simulink model "modelTest"  (R2025a)
settings: Solver=ode8  StartTime=0.0  StopTime=1000  FixedStep=0.1  RelTol=1e-3
libraries: simulink x2
settings Model: DataDictionary=Constants.sldd  PacingRate=9  Creator=levirogalla  LastModifiedBy=levirogalla
settings ModelReferenceCC: ModelReferenceMinAlgLoopOccurrences=on

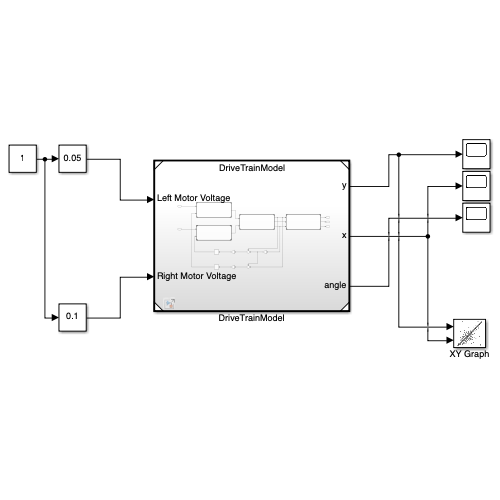
[thumbnail: Simulink's stored preview of the top-level diagram]
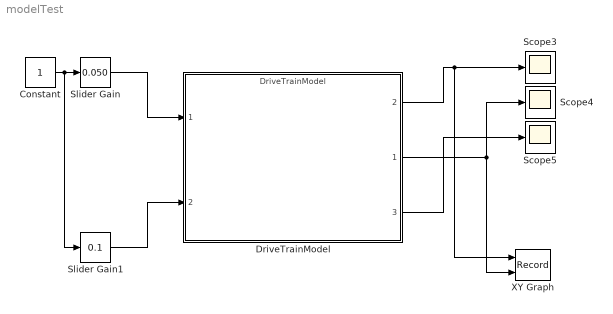
== system modelTest ==
  Constant : Constant
  DriveTrainModel : ModelReference  ModelNameDialog=DriveTrainModel.slx  SimulationMode=Normal  ModelReferenceVersion=1.6
      settings: PortSchema="{\"entries\":[{\"content\":{\"sides\":[{\"content\":{\"connectorIds\":[\"In1\",\"In2\"]},\"type\":\"ConnectorPlacement.EquallySpacedRectSide\",\"uuid\":\"dac7dafa-9168-4ba2-b9ff-6bb133c278a9\"},{\"content\":{\"connectorIds\":[\"Out2\",\"Out1\",\"Out3\"],\"side\":\"RIGHT\"},\"type\":\"ConnectorPlacement.EquallySpacedRectSide\",\"uuid\":\"23db2a58-e37d-4d01-b2f8-77513603e2c5\"},{\"content\":{\"side\":\"TOP\"},\"type\":\"ConnectorPlacement.EquallySpacedRectSide\",\"uuid\":\"ac0e75e4-011a-4388-af1c-8c3e2800fc35\"}]},\"type\":\"ConnectorPlacement.EquallySpacedConnector\",\"uuid\":\"8132e307-df65-417f-8d94-cb51f78f5789\"}],\"packageUris\":[\"http://schema.mathworks.com/mf0/Connector/R2020b\"],\"version\":\"1.0\"}"
  Scope3 : Scope
      settings: ActiveDisplayYMinimum=-125  ActiveDisplayYMaximum=1125
  Scope4 : Scope
      settings: ActiveDisplayYMinimum=-1  ActiveDisplayYMaximum=1  DataLoggingVariableName=ScopeData2
  Scope5 : Scope
      settings: ActiveDisplayYMinimum=-1  ActiveDisplayYMaximum=1  DataLoggingVariableName=ScopeData3
  Slider Gain : simulink/Math Operations/Slider Gain  gain=0.050  low=-1  high=1
  Slider Gain1 : simulink/Math Operations/Slider Gain  gain=0.1  low=-1  high=1
  XY Graph : Record  NumPorts=2.0  FileSettingsInternal="{\"entries\":[{\"content\":{\"excelSettings\":{\"content\":{},\"type\":\"Streamout.ExcelSettings\"},\"parquetSettings\":{\"content\":{},\"type\":\"Streamout.ParquetSettings\"}},\"type\":\"Streamout.FileSettingStorage\",\"uuid\":\"\"}],\"packageUris\":[\"http:\\/\\/schema.mathworks.com\\/mf0\\/streamout_blocks\\/R2020a\"],\"version\":\"1.0\"}"  FrameSettings=[0, 0]  Layout=[1 1]  SignalsInternal="{\"entries\":[{\"content\":{\"signals\":[{\"content\":{\"blockPath\":[],\"dimensions\":[1],\"domain\":\"\",\"lineColor\":\"#a2142f\",\"plots\":[ 1 ],\"port\":1,\"sid\":[\"\"],\"signalID\":1,\"signalName\":\"DriveTrainModel:2\"},\"type\":\"RecordBlkView.Signal\",\"uuid\":\"\"},{\"content\":{\"blockPath\":[],\"dimensions\":[1],\"domain\":\"\",\"lineColor\":\"#139fff\",\"plots\":[ 1 ],\"port\":2,\"sid\":[\"\"],\"signalID\":2,\"signalName\":\"DriveTrainModel:1\"},\"type\":\"RecordBlkView.Signal\",\"uuid\":\"\"}]},\"type\":\"RecordBlkView.InputSignals\",\"uuid\":\"\"}],\"packageUris\":[\"http:\\/\\/schema.mathworks.com\\/mf0\\/streamout_blocks\\/R2020a\"],\"version\":\"1.0\"}"  VisualizationBindings="{\"xyplotplugin\":{\"info\":[{\"series\":[{\"bindingParametersList\":[{\"parameter\":\"X-Axis\",\"signalID\":1,\"signalName\":\"DriveTrainModel:2\"},{\"parameter\":\"Y-Axis\",\"signalID\":2,\"signalName\":\"DriveTrainModel:1\"},{\"parameter\":\"X-Axis\",\"signalID\":1,\"signalName\":\"DriveTrainModel:2\"},{\"parameter\":\"Y-Axis\",\"signalID\":2,\"signalName\":\"DriveTrainModel:1\"}],\"seriesID\":0}],\"subplotID\":1}]}}"  CompatibilityTag=XY
  wires:
  DriveTrainModel/1 -> XY Graph/2, Scope4/1
  DriveTrainModel/3 -> Scope5/1
  Constant/1 -> Slider Gain1/1, Slider Gain/1
  Slider Gain/1 -> DriveTrainModel/1
  Slider Gain1/1 -> DriveTrainModel/2
  DriveTrainModel/2 -> XY Graph/1, Scope3/1
